simulink model "faultABCG"  (R2022b)
settings: Solver=VariableStepAuto  StartTime=0.0  StopTime=0.5  RelTol=1e-3
libraries: spsThreePhaseVIMeasurementLib x2, spsRMSLib x2, spsDistributedParametersLineLib x2, spsSequenceAnalyzerLib x2, spsThreePhaseSeriesRLCLoadLib x1, spsThreePhaseSourceLib x1, spsThreePhaseTransformerTwoWindingsLib x1, spsThreePhaseFaultLib x1, spspowerguiLib x1
settings Model: Creator=Subash  LastModifiedBy=Subash
settings DataIOCC: SaveState=on  ReturnWorkspaceOutputs=off

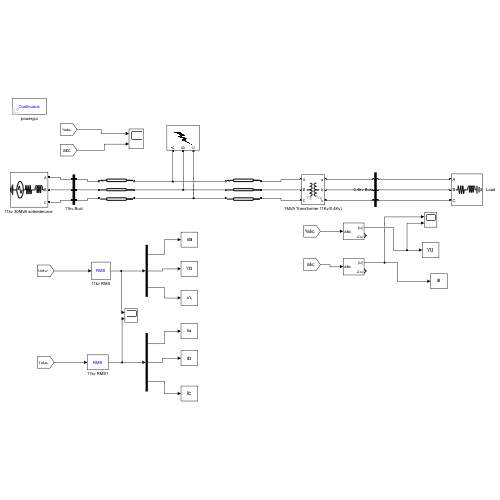
[thumbnail: Simulink's stored preview of the top-level diagram]
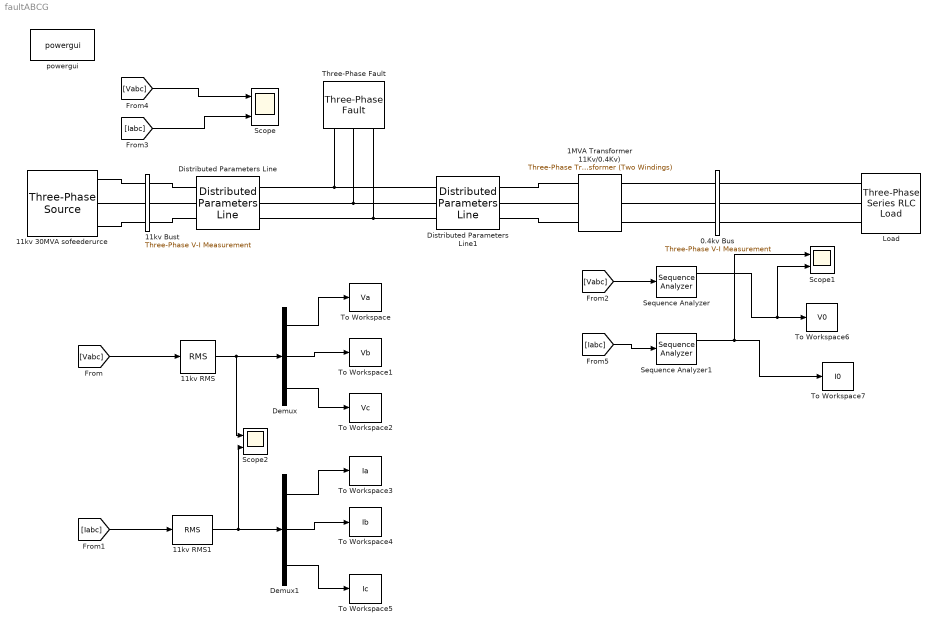
== system faultABCG ==
  " Load" : spsThreePhaseSeriesRLCLoadLib/Three-Phase Series RLC Load  LConnTagsString=A|B|C  Configuration=Y (grounded)  NominalVoltage=11000  Vabc=[1e3 1e3 1e3]  Vabcp=[1e3 1e3 1e3]  NominalFrequency=50  UnbalancedPower=off  ActivePower=11e3  InductivePower=1  CapacitivePower=0  Pabc=[10e3 9e3 11e3]  QLabc=[100 90 110]  QCabc=0  Pabcp=[10e3 9e3 11e3]  QLabcp=[100 90 110]  QCabcp=[100 90 110]  Measurements=None  LoadType=constant Z
  0.4kv Bus : spsThreePhaseVIMeasurementLib/Three-Phase V-I Measurement  VoltageMeasurement=no  SetLabelV=off  LabelV=Vabc  Vpu=off  VpuLL=off  CurrentMeasurement=no  SetLabelI=off  LabelI=Iabc  Ipu=off  Pbase=100e6  Vbase=500e3  OutputType=Complex  PhasorSimulation=off  PSBequivalent=0
  "11kv 30MVA sofeederurce " : spsThreePhaseSourceLib/Three-Phase Source  InternalConnection=Yg  VoltagePhases=off  Voltage=11e3  PhaseAngle=0  Voltage_phases=[25e3 25e3 25e3]/sqrt(3)  PhaseAngles_phases=[0 -120 +120]  Frequency=50  NonIdealSource=on  SpecifyImpedance=off  Resistance=0.8929  Inductance=16.58e-3  ShortCircuitLevel=100e6  BaseVoltage=25e3  XRratio=7  BusType=PV  Pref=30e6  Qref=0  Prefabc=[10e3, 10e3, 10e3]  Qrefabc=[0, 0, 0]  Qmin=-inf  Qmax=inf
  11kv Bust : spsThreePhaseVIMeasurementLib/Three-Phase V-I Measurement  VoltageMeasurement=phase-to-ground  SetLabelV=on  LabelV=Vabc  Vpu=off  VpuLL=off  CurrentMeasurement=yes  SetLabelI=on  LabelI=Iabc  Ipu=off  Pbase=100e6  Vbase=500e3  OutputType=Complex  PhasorSimulation=off  PSBequivalent=0
  11kv RMS : spsRMSLib/RMS  TrueRMS=on  Freq=50  RMSInit=11e3  Ts=0
  11kv RMS1 : spsRMSLib/RMS  TrueRMS=on  Freq=50  RMSInit=11e3  Ts=0
  1MVA Transformer 11Kv/0.4Kv) : spsThreePhaseTransformerTwoWindingsLib/Three-Phase Transformer (Two Windings)  Winding1Connection=Yg  Winding2Connection=Yg  CoreType=Three single-phase transformers  SetSaturation=off  Hysteresis=off  DataFile='hysteresis'  SetInitialFlux=off  Measurements=None  UNITS=pu  NominalPower=[ 250e6 , 60 ]  Winding1=[ 735e3 , 0.002 , 0.08 ]  Winding2=[ 315e3 , 0.002 , 0.08 ]  Rm=500  Lm=500  L0=0.5  Saturation=[ 0,0 ; 0.0024,1.2 ; 1.0,1.52 ]  InitialFluxes=[0.8 -0.8 0.69999]  BreakLoop=off  DiscreteSolver=Trapezoidal iterative  DataType=off  TransfoNumber=1
  Demux : Demux  Outputs=3
  Demux1 : Demux  Outputs=3
  Distributed Parameters Line : spsDistributedParametersLineLib/Distributed Parameters Line  Phases=3  Length=50  Frequency=50  Resistance=[0.01273 0.3864]  Inductance="[0.9337e-3  4.1264e-3]"  Capacitance=[12.74e-9 7.751e-9]  x1=[3.27922978200512e-12 11027.4834984327 11027.4834984327;314.159265358979 314.159265358979 314.159265358979;0.893958661638655 0.46889190324011 -1.10190442355479]  x2=[1.80529543661389e-11 11089.0531027006 11089.0531027006;314.159265358979 314.159265358979 314.159265358979;0.625255637003484 0.468372931262323 -1.10242339553257]  x3=[2.28254629454016e-13 40.7990439787102 40.7990439787106;314.159265358979 314.159265358979 314.159265358979;-0.585117128464119 0.338459033529491 -1.2323372932654]  x4=[1.03368104336393e-13 41.2133110180778 41.2133110180777;314.159265358979 314.159265358979 314.159265358979;2.43300095958087 0.543556686283164 -1.02723964051172]  x5=0.000282770783497871  V1=[3.279e-12 1.103e+04 1.103e+04;314.2 314.2 314.2;0.894 0.4689 -1.102]  V2=[1.805e-11 1.109e+04 1.109e+04;314.2 314.2 314.2;0.6253 0.4684 -1.102]  I1=[2.283e-13 40.8 40.8;314.2 314.2 314.2;-0.5851 0.3385 -1.232]  I2=[1.034e-13 41.21 41.21;314.2 314.2 314.2;2.433 0.5436 -1.027]  nHarmo=1  Measurements=None  Decoupling=off  VsMag0=0  VrMag0=0  VsAngle0=0  VrAngle0=0  IsMag0=0  IrMag0=0  IsAngle0=0  IrAngle0=0
      settings: LibrarySourceBlock=sps_lib/Power Grid Elements/Distributed Parameters Line
  Distributed Parameters Line1 : spsDistributedParametersLineLib/Distributed Parameters Line  Phases=3  Length=70  Frequency=50  Resistance=[0.01273 0.3864]  Inductance="[0.9337e-3  4.1264e-3]"  Capacitance=[12.74e-9 7.751e-9]  x1=[1.80529543661389e-11 11089.0531027006 11089.0531027006;314.159265358979 314.159265358979 314.159265358979;0.589721612360014 0.446702464698149 -1.12409386209675]  x2=[1.45020919436338e-11 11120.5760549418 11120.5760549418;314.159265358979 314.159265358979 314.159265358979;0.727597240921128 0.4462161057795 -1.1245802210154]  x3=[1.56936056748742e-14 40.7816260727145 40.7816260727144;314.159265358979 314.159265358979 314.159265358979;3.01722356733765 0.370757130598738 -1.20003919619617]  x4=[6.55626720188216e-14 41.1722015741792 41.1722015741795;314.159265358979 314.159265358979 314.159265358979;-1.85542924853397 0.445893419370665 -1.12490290742422]  x5=0.00039587909689702  V1=[1.805e-11 1.109e+04 1.109e+04;314.2 314.2 314.2;0.5897 0.4467 -1.124]  V2=[1.45e-11 1.112e+04 1.112e+04;314.2 314.2 314.2;0.7276 0.4462 -1.125]  I1=[1.569e-14 40.78 40.78;314.2 314.2 314.2;3.017 0.3708 -1.2]  I2=[6.556e-14 41.17 41.17;314.2 314.2 314.2;-1.855 0.4459 -1.125]  nHarmo=1  Measurements=None  Decoupling=off  VsMag0=0  VrMag0=0  VsAngle0=0  VrAngle0=0  IsMag0=0  IrMag0=0  IsAngle0=0  IrAngle0=0
      settings: LibrarySourceBlock=sps_lib/Power Grid Elements/Distributed Parameters Line
  Scope : Scope  NumInputPorts=2
  Scope1 : Scope  NumInputPorts=2
  Scope2 : Scope  NumInputPorts=2
  Sequence Analyzer : spsSequenceAnalyzerLib/Sequence Analyzer  Freq=50  n=1  seq=Positive Negative Zero  InInit=[1, 0]  Ts=0
      settings: LibrarySourceBlock=sps_lib/Sensors and Measurements/Sequence Analyzer
  Sequence Analyzer1 : spsSequenceAnalyzerLib/Sequence Analyzer  Freq=50  n=1  seq=Positive Negative Zero  InInit=[1, 0]  Ts=0
      settings: LibrarySourceBlock=sps_lib/Sensors and Measurements/Sequence Analyzer
  Three-Phase Fault : spsThreePhaseFaultLib/Three-Phase Fault  InitialStates=0  FaultA=on  FaultB=on  FaultC=on  GroundFault=on  SwitchTimes=[0.2 0.3]  External=off  SwitchStatus=NaN  FaultResistance=0.001  GroundResistance=0.01  SnubberResistance=1e6  SnubberCapacitance=inf  Measurements=Fault voltages and currents
  To Workspace : ToWorkspace  VariableName=Va  SaveFormat=Timeseries  SampleTime=-1
  To Workspace1 : ToWorkspace  VariableName=Vb  SaveFormat=Timeseries  SampleTime=-1
  To Workspace2 : ToWorkspace  VariableName=Vc  SaveFormat=Timeseries  SampleTime=-1
  To Workspace3 : ToWorkspace  VariableName=Ia  SaveFormat=Timeseries  SampleTime=-1
  To Workspace4 : ToWorkspace  VariableName=Ib  SaveFormat=Timeseries  SampleTime=-1
  To Workspace5 : ToWorkspace  VariableName=Ic  SaveFormat=Timeseries  SampleTime=-1
  To Workspace6 : ToWorkspace  VariableName=V0  SaveFormat=Timeseries  SampleTime=-1
  To Workspace7 : ToWorkspace  VariableName=I0  SaveFormat=Timeseries  SampleTime=-1
  powergui : spspowerguiLib/powergui  Priority=1  SimulationMode=Continuous  SampleTime=50e-6  frequency=60  Iterations=50  frequencyindice=50  Pbase=100e6  ErrMax=1e-4  UnitsV=kV  UnitsW=MW  buscounter=0  FunctionMessages=off  echomessages=off  EnableUseOfTLC=off  CurrentSourceSwitches=off  DisableSnubberDevices=off  DisableRonSwitches=off  DisableVfSwitches=off  DisplayEquations=off  AutomaticDiscreteSolvers=off  SolverType=Tustin/Backward Euler (TBE)  Interpol=off  ExternalGateDelay=off  methode=off  Ts=100  x0status=blocks  SPID=on  SwTol=0  HookPort=off  NonlinearTolerance=1e-4  nMaxIteration=100  ContinueOnMaxIteration=off  RestoreLinks=warning  ResistiveCurrentMeasurement=off  Frange=[0:2:500]  Ylog=off  Xlog=on  ShowGrid=off  save=off  variable=ZData  structure=0  ZoomFFT=off  StartTime=0.0  cycles=1  DisplayStyle=1  fundamental=60  FreqAxis=off  MaxFrequency=1000  frequencyindicesteady=1  RmsSteady=1  display=off
  wires:
  Sequence Analyzer1/1 -> Scope1/1, To Workspace7/1
  [Iabc] -> Scope/2
  [Vabc] -> Scope/1
  Demux/2 -> To Workspace1/1
  Demux1/3 -> To Workspace5/1
  Demux/3 -> To Workspace2/1
  11kv RMS1/1 -> Scope2/2, Demux1/1
  11kv RMS/1 -> Scope2/1, Demux/1
  Demux/1 -> To Workspace/1
  Demux1/1 -> To Workspace3/1
  Demux1/2 -> To Workspace4/1
  Sequence Analyzer/1 -> Scope1/2, To Workspace6/1
  [Vabc] -> Sequence Analyzer/1
  [Iabc] -> 11kv RMS1/1
  [Vabc] -> 11kv RMS/1
  [Iabc] -> Sequence Analyzer1/1
  connections:
  Three-Phase Fault/LConn3 -- Distributed Parameters Line1/LConn3 -- Distributed Parameters Line/RConn3
  Distributed Parameters Line/RConn1 -- Distributed Parameters Line1/LConn1 -- Three-Phase Fault/LConn1
  Three-Phase Fault/LConn2 -- Distributed Parameters Line1/LConn2 -- Distributed Parameters Line/RConn2
  " Load"/LConn2 -- 0.4kv Bus/RConn2
  Distributed Parameters Line/LConn3 -- 11kv Bust/RConn3
  " Load"/LConn1 -- 0.4kv Bus/RConn1
  "11kv 30MVA sofeederurce "/RConn1 -- 11kv Bust/LConn1
  Distributed Parameters Line1/RConn1 -- 1MVA Transformer 11Kv/0.4Kv)/LConn1
  Distributed Parameters Line/LConn1 -- 11kv Bust/RConn1
  Distributed Parameters Line/LConn2 -- 11kv Bust/RConn2
  "11kv 30MVA sofeederurce "/RConn2 -- 11kv Bust/LConn2
  Distributed Parameters Line1/RConn2 -- 1MVA Transformer 11Kv/0.4Kv)/LConn2
  1MVA Transformer 11Kv/0.4Kv)/RConn3 -- 0.4kv Bus/LConn3
  " Load"/LConn3 -- 0.4kv Bus/RConn3
  1MVA Transformer 11Kv/0.4Kv)/RConn2 -- 0.4kv Bus/LConn2
  Distributed Parameters Line1/RConn3 -- 1MVA Transformer 11Kv/0.4Kv)/LConn3
  "11kv 30MVA sofeederurce "/RConn3 -- 11kv Bust/LConn3
  1MVA Transformer 11Kv/0.4Kv)/RConn1 -- 0.4kv Bus/LConn1
